simulink model "trans3"  (Simulink 8.5)
settings: Solver=ode15s  SolverMode=SingleTasking  StartTime=0.0  StopTime=0.4  RelTol=1e-3  AbsTol=1e-6
undefined symbols (not defined in the file or in its folder): D1, Delta
libraries: powerlib x59
settings Model: Creator=Dr. Lotfifard  LastModifiedBy=PC
settings DataIOCC: LimitDataPoints=off
settings OptimizationCC: BlockReduction=off  BooleanDataType=off
settings DebuggingCC: SaveWithParameterizedLinksMsg=none  SignalResolutionControl=TryResolveAllWithWarning  MultiTaskDSMMsg=warning  MultiTaskCondExecSysMsg=none  FcnCallInpInsideContextMsg=UseLocalSettings  StrictBusMsg=None
settings HardwareCC: TargetUnknown=on

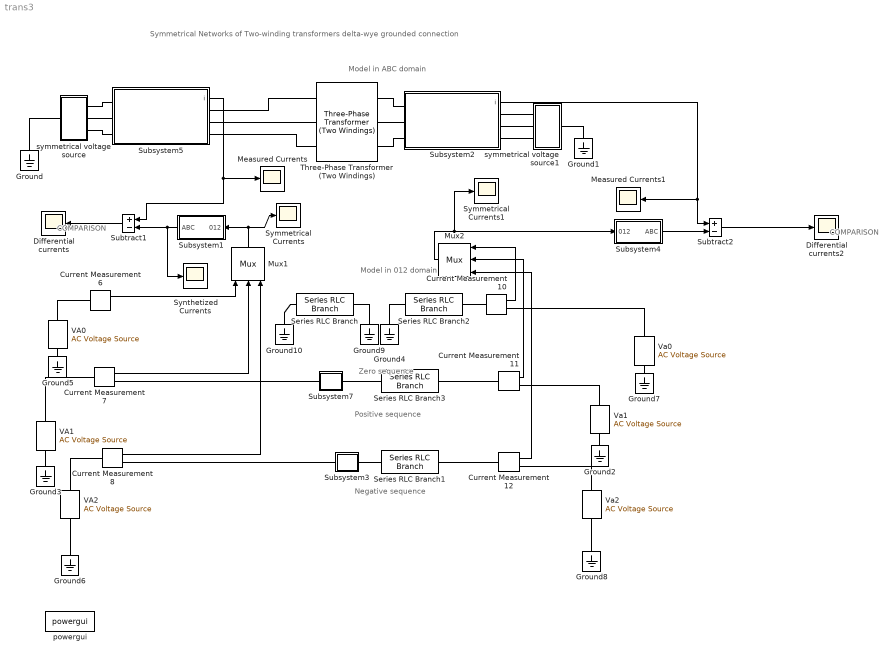
== system trans3 ==
  note: Symmetrical Networks of Two-winding transformers
      | delta-wye grounded connection
  note: Model in ABC domain
  note: Model
      | in 012 domain
  note: Positive sequence
  note: Negative sequence
  note: COMPARISON
  note: COMPARISON
  note: Zero sequence
  Current Measurement{6..8,10..12} (6 alike) : powerlib/Measurements/Current Measurement  PhasorSimulation=off  OutputType=Complex  PSBequivalent=0
  Differential currents : Scope
      settings: TickLabels=on  TimeRange=0.1  YMin=-1000  YMax=4000  SaveName=ScopeData2
  Differential currents2 : Scope
      settings: TickLabels=on  TimeRange=0.1  YMin=-1000  YMax=4000
  Ground{,1..10} (11 alike) : powerlib/Elements/Ground  LConnTagsString=a
  Measured Currents : Scope
      settings: TickLabels=on  TimeRange=0.1  YMin=-3  YMax=3  SaveName=ScopeData3
  Measured Currents1 : Scope
      settings: TickLabels=on  TimeRange=0.1  YMin=-3  YMax=3  SaveName=ScopeData4
  Mux1 : Mux  Inputs=3
  Mux2 : Mux  Inputs=3
  Series RLC Branch{,1..3} (4 alike) : powerlib/Elements/Series RLC Branch  LConnTagsString=__new0  RConnTagsString=__new0  BranchType=RL  Resistance=1  Inductance=1e-3  SetiL0=off  InitialCurrent=0  Capacitance=1e-6  Setx0=off  InitialVoltage=0  Measurements=None
  Subsystem1 : Subsystem
  Subsystem2 : Subsystem
      mask Display: disp('Current\nMeasurements')
  Subsystem3 : Subsystem  mask{k=315/13.8, phase1=1}
      mask prompts: k "Voltage Ratio(Primary/Secondary)"; phase1 "Phase Shift Vector"
      mask help:
      | This is part of the positive sequence network of the transformer.
      | The parameter Phase Shift Vector denotes that the secondary side voltage lags the primary side voltage by Vector*30 degrees
      mask init:
      | phase=phase1*30;
      mask TypeOptions phase1: 1 | 3 | 5 | 7 | 9 | 11
      mask Display: plot(0,0,100,100,[40,32,27,24,22,21,22,24,28,32,40,48,52,56,58,60,58,56,53,48,40],[70,68,65,60,56,49,43,39,35,32,30,32,35,39,43,49,56,61,65,68,70],[60,58,54,51,47,45,43,41,43,45,53,60,68,72,76,78,80,78,76,72,68,60],[70,70,70,68,65,61,56,50,43,38,32,30,32,33,38,43,49,57,62,65,68,70])
  Subsystem4 : Subsystem
  Subsystem5 : Subsystem
      mask Display: disp('Current\nMeasurements')
  Subsystem7 : Subsystem  mask{k=315/13.8, phase1=1}
      mask prompts: k "Voltage Ratio(Primary/Secondary)"; phase1 "Phase Shift Vector"
      mask help:
      | This is part of the positive sequence network of the transformer.
      | The parameter Phase Shift Vector denotes that the secondary side voltage lags the primary side voltage by Vector*30 degrees
      mask init:
      | phase=phase1*30;
      mask TypeOptions phase1: 1 | 3 | 5 | 7 | 9 | 11
      mask Display: plot(0,0,100,100,[40,32,27,24,22,21,22,24,28,32,40,48,52,56,58,60,58,56,53,48,40],[70,68,65,60,56,49,43,39,35,32,30,32,35,39,43,49,56,61,65,68,70],[60,58,54,51,47,45,43,41,43,45,53,60,68,72,76,78,80,78,76,72,68,60],[70,70,70,68,65,61,56,50,43,38,32,30,32,33,38,43,49,57,62,65,68,70])
  Subtract1 : Sum  Inputs=+-  SaturateOnIntegerOverflow=on  InputSameDT=on  OutDataTypeStr=Inherit: Same as first input
  Subtract2 : Sum  Inputs=+-  SaturateOnIntegerOverflow=on  InputSameDT=on  OutDataTypeStr=Inherit: Same as first input
  Symmetrical Currents : Scope
      settings: TickLabels=on  TimeRange=0.1  YMin=-3  YMax=3  SaveName=ScopeData5
  Symmetrical Currents1 : Scope
      settings: TickLabels=on  TimeRange=0.1  YMin=-3  YMax=3  SaveName=ScopeData6
  Synthetized Currents : Scope
      settings: TickLabels=on  TimeRange=0.1  YMin=-3  YMax=3
  Three-Phase Transformer (Two Windings) : powerlib/Elements/Three-Phase Transformer (Two Windings)  Winding1Connection=Delta (D1)  Winding2Connection=Yg  CoreType=Three single-phase transformers  SetSaturation=off  Hysteresis=off  DataFile='hysteresis'  SetInitialFlux=off  Measurements=None  UNITS=pu  NominalPower=[ 300e6 60 ]  Winding1="[ 315e3 0.01  0.1 ]"  Winding2=[ 13.8e3 0.01 0.1]  Rm=500  Lm=500  L0=0.5  Saturation=[ 0,0 ; 0.0024,1.2 ; 1.0,1.52 ]  InitialFluxes=[ 0.8 , -0.8 , 0.7 ]  MoreParameters=off  BreakLoop=off  DataType=off  TransfoNumber=1
  VA0 : powerlib/Electrical Sources/AC Voltage Source  Amplitude=0.031  Phase=-78  Frequency=60  SampleTime=0  Measurements=None
  VA1 : powerlib/Electrical Sources/AC Voltage Source  Amplitude=0.963  Phase=-6.56  Frequency=60  SampleTime=0  Measurements=None
  VA2 : powerlib/Electrical Sources/AC Voltage Source  Amplitude=0.145  Phase=75.41  Frequency=60  SampleTime=0  Measurements=None
  Va0 : powerlib/Electrical Sources/AC Voltage Source  Amplitude=0.031  Phase=-78  Frequency=60  SampleTime=0  Measurements=None
  Va1 : powerlib/Electrical Sources/AC Voltage Source  Amplitude=0.963  Phase=-6.56  Frequency=60  SampleTime=0  Measurements=None
  Va2 : powerlib/Electrical Sources/AC Voltage Source  Amplitude=0.145  Phase=75.41  Frequency=60  SampleTime=0  Measurements=None
  powergui : powerlib/powergui  SimulationMode=Continuous  SolverType=Tustin/Backward Euler (TBE)  SampleTime=0  frequency=60  SPID=off  DisableSnubberDevices=off  DisableRonSwitches=off  DisableVfSwitches=off  SwTol=0  DisplayEquations=off  Interpol=off  methode=off  Ts=0  FunctionMessages=off  echomessages=off  HookPort=off  EnableUseOfTLC=off  x0status=blocks  frequencyindice=60  Pbase=100e6  ErrMax=1e-4  Iterations=50  UnitsV=kV  UnitsW=MW  buscounter=0  RestoreLinks=warning  ResistiveCurrentMeasurement=off  Frange=[0:2:500]  Ylog=off  Xlog=on  ShowGrid=off  save=off  variable=ZData  structure=0  ZoomFFT=on  StartTime=0.0  cycles=1  DisplayStyle=1  fundamental=60  FreqAxis=off  MaxFrequency=1000  frequencyindicesteady=1  RmsSteady=1  display=off
  symmetrical voltage source : Subsystem
  symmetrical voltage source1 : Subsystem
  wires:
  Current Measurement6/1 -> Mux1/1
  Current Measurement7/1 -> Mux1/2
  Current Measurement8/1 -> Mux1/3
  Subsystem4/1(ABC) -> Subtract2/2
  Subtract1/1 -> Differential currents/1
  Subsystem5/1(i) -> Subtract1/1, Measured Currents/1
  Mux1/1 -> Subsystem1/1(012), Symmetrical Currents/1
  Mux2/1 -> Subsystem4/1(012), Symmetrical Currents1/1
  Subsystem2/1(i) -> Subtract2/1, Measured Currents1/1
  Subsystem1/1(ABC) -> Subtract1/2, Synthetized Currents/1
  Current Measurement12/1 -> Mux2/3
  Current Measurement11/1 -> Mux2/2
  Current Measurement10/1 -> Mux2/1
  Subtract2/1 -> Differential currents2/1
  connections:
  Subsystem3/LConn1 -- Current Measurement8/RConn1
  Subsystem3/RConn1 -- Series RLC Branch1/LConn1
  Series RLC Branch3/LConn1 -- Subsystem7/RConn1
  Subsystem7/LConn1 -- Current Measurement7/RConn1
  Series RLC Branch3/RConn1 -- Current Measurement11/LConn1
  Series RLC Branch1/RConn1 -- Current Measurement12/LConn1
  Series RLC Branch/RConn1 -- Ground9/LConn1
  Series RLC Branch2/LConn1 -- Ground4/LConn1
  symmetrical voltage source/LConn1 -- Ground/LConn1
  symmetrical voltage source1/RConn1 -- Subsystem2/RConn1
  Subsystem2/RConn2 -- symmetrical voltage source1/RConn2
  symmetrical voltage source1/RConn3 -- Subsystem2/RConn3
  Ground1/LConn1 -- symmetrical voltage source1/LConn1
  Three-Phase Transformer (Two Windings)/RConn2 -- Subsystem2/LConn2
  Subsystem2/LConn1 -- Three-Phase Transformer (Two Windings)/RConn1
  Subsystem2/LConn3 -- Three-Phase Transformer (Two Windings)/RConn3
  Three-Phase Transformer (Two Windings)/LConn2 -- Subsystem5/RConn2
  Three-Phase Transformer (Two Windings)/LConn1 -- Subsystem5/RConn1
  Three-Phase Transformer (Two Windings)/LConn3 -- Subsystem5/RConn3
  Subsystem5/LConn2 -- symmetrical voltage source/RConn2
  Subsystem5/LConn1 -- symmetrical voltage source/RConn1
  Subsystem5/LConn3 -- symmetrical voltage source/RConn3
  Ground5/LConn1 -- VA0/LConn1
  Ground3/LConn1 -- VA1/LConn1
  Ground6/LConn1 -- VA2/LConn1
  Current Measurement6/LConn1 -- VA0/RConn1
  Current Measurement7/LConn1 -- VA1/RConn1
  Current Measurement8/LConn1 -- VA2/RConn1
  Ground7/LConn1 -- Va0/LConn1
  Ground2/LConn1 -- Va1/LConn1
  Ground8/LConn1 -- Va2/LConn1
  Current Measurement11/RConn1 -- Va1/RConn1
  Va2/RConn1 -- Current Measurement12/RConn1
  Va0/RConn1 -- Current Measurement10/RConn1
  Series RLC Branch2/RConn1 -- Current Measurement10/LConn1
  Ground10/LConn1 -- Series RLC Branch/LConn1

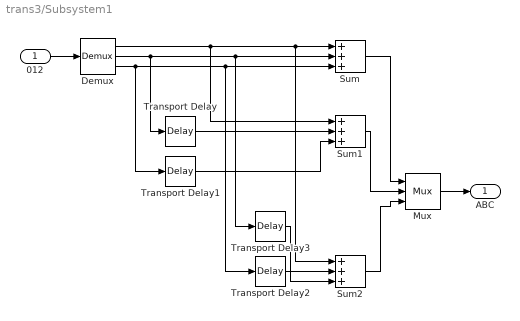
== system trans3/Subsystem1 ==
  012 : Inport
  Demux : Demux  Outputs=3
  Mux : Mux  Inputs=3
  Sum : Sum  Inputs=+++  SaturateOnIntegerOverflow=on  InputSameDT=on  OutDataTypeStr=Inherit: Same as first input
  Sum1 : Sum  Inputs=+++  SaturateOnIntegerOverflow=on  InputSameDT=on  OutDataTypeStr=Inherit: Same as first input
  Sum2 : Sum  Inputs=+++  SaturateOnIntegerOverflow=on  InputSameDT=on  OutDataTypeStr=Inherit: Same as first input
  Transport Delay : TransportDelay  DelayTime=1/(3*60)
  Transport Delay1 : TransportDelay  DelayTime=2/(3*60)
  Transport Delay2 : TransportDelay  DelayTime=1/(3*60)
  Transport Delay3 : TransportDelay  DelayTime=2/(3*60)
  ABC : Outport  InitialOutput=0
  wires:
  012/1 -> Demux/1
  Sum1/1 -> Mux/2
  Sum/1 -> Mux/1
  Mux/1 -> ABC/1
  Sum2/1 -> Mux/3
  Demux/2 -> Transport Delay/1, Sum/2, Transport Delay3/1
  Demux/3 -> Transport Delay1/1, Sum/3, Transport Delay2/1
  Demux/1 -> Sum1/1, Sum/1, Sum2/1
  Transport Delay/1 -> Sum1/2
  Transport Delay1/1 -> Sum1/3
  Transport Delay2/1 -> Sum2/3
  Transport Delay3/1 -> Sum2/2

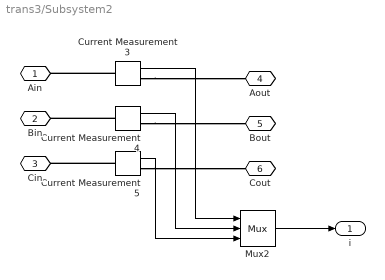
== system trans3/Subsystem2 ==
  Current Measurement3 : powerlib/Measurements/Current Measurement  PhasorSimulation=off  OutputType=Complex  PSBequivalent=0
  Current Measurement4 : powerlib/Measurements/Current Measurement  PhasorSimulation=off  OutputType=Complex  PSBequivalent=0
  Current Measurement5 : powerlib/Measurements/Current Measurement  PhasorSimulation=off  OutputType=Complex  PSBequivalent=0
  Mux2 : Mux  Inputs=3
  Ain : PMIOPort  Port=1  Side=Left
  Bin : PMIOPort  Port=2  Side=Left
  Cin : PMIOPort  Port=3  Side=Left
  Aout : PMIOPort  Port=4  Side=Right
  Bout : PMIOPort  Port=5  Side=Right
  Cout : PMIOPort  Port=6  Side=Right
  i : Outport  InitialOutput=0
  wires:
  Current Measurement3/1 -> Mux2/1
  Current Measurement4/1 -> Mux2/2
  Current Measurement5/1 -> Mux2/3
  Mux2/1 -> i/1
  connections:
  Current Measurement3/LConn1 -- Ain/RConn1
  Current Measurement4/LConn1 -- Bin/RConn1
  Current Measurement5/LConn1 -- Cin/RConn1
  Current Measurement3/RConn1 -- Aout/RConn1
  Current Measurement4/RConn1 -- Bout/RConn1
  Current Measurement5/RConn1 -- Cout/RConn1

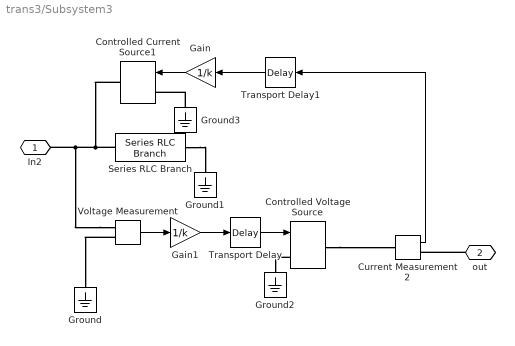
== system trans3/Subsystem3 ==
  Controlled Current Source1 : powerlib/Electrical Sources/Controlled Current Source  Tag=PoWeRsYsTeMbLoCk  Initialize=on  Source_Type=AC  Amplitude=0  Phase=0  Frequency=0  Measurements=None
  Controlled Voltage Source : powerlib/Electrical Sources/Controlled Voltage Source  Tag=PoWeRsYsTeMbLoCk  Initialize=on  Source_Type=AC  Amplitude=0  Phase=0  Frequency=0  Measurements=None
  Current Measurement2 : powerlib/Measurements/Current Measurement  Tag=PoWeRsYsTeMmEaSuReMeNt  PhasorSimulation=off  OutputType=Complex  PSBequivalent=0
  Gain : Gain  Gain=1/k  SaturateOnIntegerOverflow=on  OutDataTypeStr=Inherit: Same as input  ParamDataTypeStr=Inherit: Same as input
  Gain1 : Gain  Gain=1/k  SaturateOnIntegerOverflow=on  OutDataTypeStr=Inherit: Same as input  ParamDataTypeStr=Inherit: Same as input
  Ground{,1..3} (4 alike) : powerlib/Elements/Ground  LConnTagsString=a
  Series RLC Branch : powerlib/Elements/Series RLC Branch  LConnTagsString=__new0  RConnTagsString=__new0  BranchType=RL  Resistance=1  Inductance=1e-3  SetiL0=off  InitialCurrent=0  Capacitance=1e-6  Setx0=off  InitialVoltage=0  Measurements=None
  Transport Delay : TransportDelay  DelayTime=phase/360*(1/60)
  Transport Delay1 : TransportDelay  DelayTime=(360-phase)/360*(1/60)
  Voltage Measurement : powerlib/Measurements/Voltage Measurement  Tag=PoWeRsYsTeMmEaSuReMeNt  PhasorSimulation=off  OutputType=Complex  PSBequivalent=0
  In2 : PMIOPort  Port=1  Side=Left
  out : PMIOPort  Port=2  Side=Right
  wires:
  Current Measurement2/1 -> Transport Delay1/1
  Transport Delay/1 -> Controlled Voltage Source/1
  Gain1/1 -> Transport Delay/1
  Voltage Measurement/1 -> Gain1/1
  Transport Delay1/1 -> Gain/1
  Gain/1 -> Controlled Current Source1/1
  connections:
  out/RConn1 -- Current Measurement2/RConn1
  Voltage Measurement/LConn2 -- Ground/LConn1
  Voltage Measurement/LConn1 -- Series RLC Branch/LConn1 -- Controlled Current Source1/RConn1 -- In2/RConn1
  Series RLC Branch/RConn1 -- Ground1/LConn1
  Controlled Voltage Source/LConn1 -- Ground2/LConn1
  Ground3/LConn1 -- Controlled Current Source1/LConn1
  Controlled Voltage Source/RConn1 -- Current Measurement2/LConn1

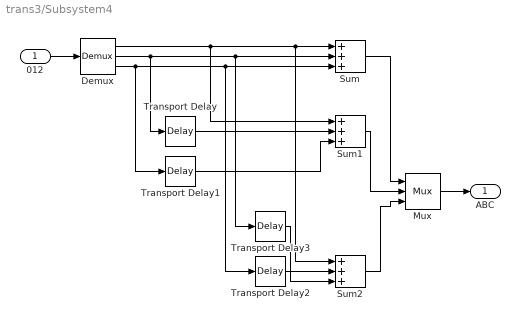
== system trans3/Subsystem4 ==
  012 : Inport
  Demux : Demux  Outputs=3
  Mux : Mux  Inputs=3
  Sum : Sum  Inputs=+++  SaturateOnIntegerOverflow=on  InputSameDT=on  OutDataTypeStr=Inherit: Same as first input
  Sum1 : Sum  Inputs=+++  SaturateOnIntegerOverflow=on  InputSameDT=on  OutDataTypeStr=Inherit: Same as first input
  Sum2 : Sum  Inputs=+++  SaturateOnIntegerOverflow=on  InputSameDT=on  OutDataTypeStr=Inherit: Same as first input
  Transport Delay : TransportDelay  DelayTime=1/(3*60)
  Transport Delay1 : TransportDelay  DelayTime=2/(3*60)
  Transport Delay2 : TransportDelay  DelayTime=1/(3*60)
  Transport Delay3 : TransportDelay  DelayTime=2/(3*60)
  ABC : Outport  InitialOutput=0
  wires:
  012/1 -> Demux/1
  Sum1/1 -> Mux/2
  Sum/1 -> Mux/1
  Mux/1 -> ABC/1
  Sum2/1 -> Mux/3
  Demux/2 -> Transport Delay/1, Sum/2, Transport Delay3/1
  Demux/3 -> Transport Delay1/1, Sum/3, Transport Delay2/1
  Demux/1 -> Sum1/1, Sum/1, Sum2/1
  Transport Delay/1 -> Sum1/2
  Transport Delay1/1 -> Sum1/3
  Transport Delay2/1 -> Sum2/3
  Transport Delay3/1 -> Sum2/2

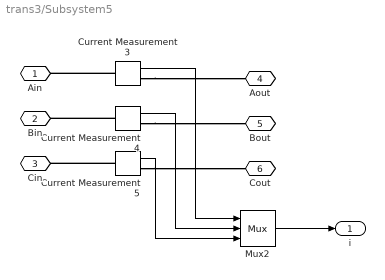
== system trans3/Subsystem5 ==
  Current Measurement3 : powerlib/Measurements/Current Measurement  PhasorSimulation=off  OutputType=Complex  PSBequivalent=0
  Current Measurement4 : powerlib/Measurements/Current Measurement  PhasorSimulation=off  OutputType=Complex  PSBequivalent=0
  Current Measurement5 : powerlib/Measurements/Current Measurement  PhasorSimulation=off  OutputType=Complex  PSBequivalent=0
  Mux2 : Mux  Inputs=3
  Ain : PMIOPort  Port=1  Side=Left
  Bin : PMIOPort  Port=2  Side=Left
  Cin : PMIOPort  Port=3  Side=Left
  Aout : PMIOPort  Port=4  Side=Right
  Bout : PMIOPort  Port=5  Side=Right
  Cout : PMIOPort  Port=6  Side=Right
  i : Outport  InitialOutput=0
  wires:
  Current Measurement3/1 -> Mux2/1
  Current Measurement4/1 -> Mux2/2
  Current Measurement5/1 -> Mux2/3
  Mux2/1 -> i/1
  connections:
  Current Measurement3/LConn1 -- Ain/RConn1
  Current Measurement4/LConn1 -- Bin/RConn1
  Current Measurement5/LConn1 -- Cin/RConn1
  Current Measurement3/RConn1 -- Aout/RConn1
  Current Measurement4/RConn1 -- Bout/RConn1
  Current Measurement5/RConn1 -- Cout/RConn1

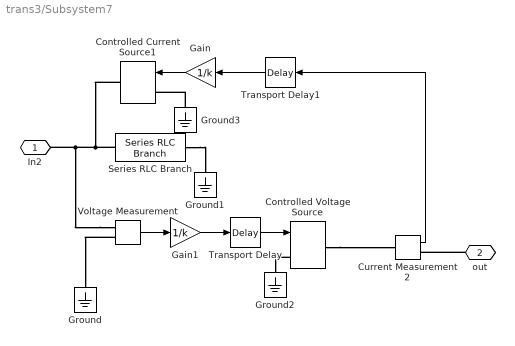
== system trans3/Subsystem7 ==
  Controlled Current Source1 : powerlib/Electrical Sources/Controlled Current Source  Tag=PoWeRsYsTeMbLoCk  Initialize=on  Source_Type=AC  Amplitude=0  Phase=0  Frequency=0  Measurements=None
  Controlled Voltage Source : powerlib/Electrical Sources/Controlled Voltage Source  Tag=PoWeRsYsTeMbLoCk  Initialize=on  Source_Type=AC  Amplitude=0  Phase=0  Frequency=0  Measurements=None
  Current Measurement2 : powerlib/Measurements/Current Measurement  Tag=PoWeRsYsTeMmEaSuReMeNt  PhasorSimulation=off  OutputType=Complex  PSBequivalent=0
  Gain : Gain  Gain=1/k  SaturateOnIntegerOverflow=on  OutDataTypeStr=Inherit: Same as input  ParamDataTypeStr=Inherit: Same as input
  Gain1 : Gain  Gain=1/k  SaturateOnIntegerOverflow=on  OutDataTypeStr=Inherit: Same as input  ParamDataTypeStr=Inherit: Same as input
  Ground{,1..3} (4 alike) : powerlib/Elements/Ground  LConnTagsString=a
  Series RLC Branch : powerlib/Elements/Series RLC Branch  LConnTagsString=__new0  RConnTagsString=__new0  BranchType=RL  Resistance=1  Inductance=1e-3  SetiL0=off  InitialCurrent=0  Capacitance=1e-6  Setx0=off  InitialVoltage=0  Measurements=None
  Transport Delay : TransportDelay  DelayTime=(360-phase)/360*(1/60)
  Transport Delay1 : TransportDelay  DelayTime=phase/360*(1/60)
  Voltage Measurement : powerlib/Measurements/Voltage Measurement  Tag=PoWeRsYsTeMmEaSuReMeNt  PhasorSimulation=off  OutputType=Complex  PSBequivalent=0
  In2 : PMIOPort  Port=1  Side=Left
  out : PMIOPort  Port=2  Side=Right
  wires:
  Current Measurement2/1 -> Transport Delay1/1
  Transport Delay/1 -> Controlled Voltage Source/1
  Gain1/1 -> Transport Delay/1
  Voltage Measurement/1 -> Gain1/1
  Transport Delay1/1 -> Gain/1
  Gain/1 -> Controlled Current Source1/1
  connections:
  out/RConn1 -- Current Measurement2/RConn1
  Voltage Measurement/LConn2 -- Ground/LConn1
  Voltage Measurement/LConn1 -- Series RLC Branch/LConn1 -- Controlled Current Source1/RConn1 -- In2/RConn1
  Series RLC Branch/RConn1 -- Ground1/LConn1
  Controlled Voltage Source/LConn1 -- Ground2/LConn1
  Ground3/LConn1 -- Controlled Current Source1/LConn1
  Controlled Voltage Source/RConn1 -- Current Measurement2/LConn1

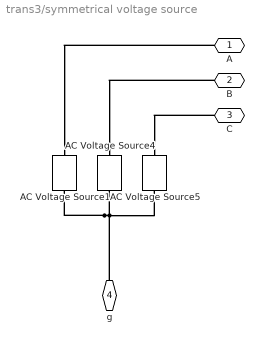
== system trans3/symmetrical voltage source ==
  AC Voltage Source1 : powerlib/Electrical Sources/AC Voltage Source  Amplitude=315e3/sqrt(3)*sqrt(2)  Phase=0  Frequency=60  SampleTime=0  Measurements=None
  AC Voltage Source4 : powerlib/Electrical Sources/AC Voltage Source  Amplitude=315e3/sqrt(3)*sqrt(2)  Phase=-80  Frequency=60  SampleTime=0  Measurements=None
  AC Voltage Source5 : powerlib/Electrical Sources/AC Voltage Source  Amplitude=315e3/sqrt(3)*sqrt(2)  Phase=60  Frequency=60  SampleTime=0  Measurements=None
  A : PMIOPort  Port=1  Side=Right
  B : PMIOPort  Port=2  Side=Right
  C : PMIOPort  Port=3  Side=Right
  g : PMIOPort  Port=4  Side=Left
  connections:
  AC Voltage Source4/LConn1 -- AC Voltage Source5/LConn1 -- AC Voltage Source1/LConn1 -- g/RConn1
  B/RConn1 -- AC Voltage Source4/RConn1
  A/RConn1 -- AC Voltage Source1/RConn1
  C/RConn1 -- AC Voltage Source5/RConn1

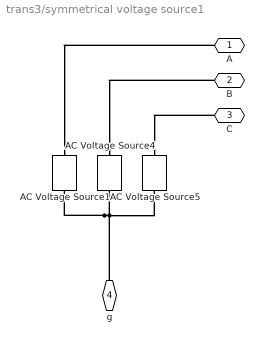
== system trans3/symmetrical voltage source1 ==
  AC Voltage Source1 : powerlib/Electrical Sources/AC Voltage Source  Amplitude=315e3/sqrt(3)*sqrt(2)  Phase=0  Frequency=60  SampleTime=0  Measurements=None
  AC Voltage Source4 : powerlib/Electrical Sources/AC Voltage Source  Amplitude=315e3/sqrt(3)*sqrt(2)  Phase=-80  Frequency=60  SampleTime=0  Measurements=None
  AC Voltage Source5 : powerlib/Electrical Sources/AC Voltage Source  Amplitude=315e3/sqrt(3)*sqrt(2)  Phase=60  Frequency=60  SampleTime=0  Measurements=None
  A : PMIOPort  Port=1  Side=Right
  B : PMIOPort  Port=2  Side=Right
  C : PMIOPort  Port=3  Side=Right
  g : PMIOPort  Port=4  Side=Left
  connections:
  AC Voltage Source5/LConn1 -- AC Voltage Source1/LConn1 -- g/RConn1 -- AC Voltage Source4/LConn1
  B/RConn1 -- AC Voltage Source4/RConn1
  A/RConn1 -- AC Voltage Source1/RConn1
  C/RConn1 -- AC Voltage Source5/RConn1
